simulink library "simetranss"  (R2024b)
settings: Solver=VariableStepAuto  StartTime=0.0  StopTime=10.0  RelTol=1e-3
PostLoadFcn:
  | Ts=1e-6
InitFcn:
  | Ts=1e-6
undefined symbols (not defined in the file): C, C_601, C_603, C_606, CC, Csnu, Csnubber, DiscIntNeverNeededParam, DPL, DPL1ph, FluxTable, ft2km, gcbh, h, Half, Imap2, L, L_601, L_603, L_606, Lbase, LpejoSw, Newton, R_601, R_603, R_606, Raphson, ResistanceM, Roff, Ron, RotorAngles, Rsnu, Rsnubber, Rt4, SampleTime, simetran, sps, sps_rtmsupport, StatorCurrents, T_2wind_ratio, T_Lpu, T_Lpu_pri, T_Rpu, T_Rpu_pri, T_Vpri, T_Vpri_15comp, T_Vsec, Ti, Ts_Power, Z, Zbase, Zm
libraries: fl_lib x248, ee_lib x146, nesl_utility x122, $bdroot x29, simulink x15, eeGeneralControl x2, spsStairGeneratorLib x2, artemis x1
(part 1 of 12)
Description:
  | Collection of custom SimScape real-time models.
settings Model: ModifiedByFormat=KD  Creator=Kyle Diller  LastModifiedBy=KD

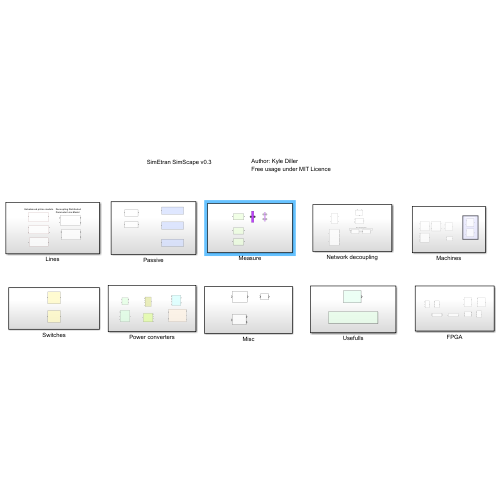
[thumbnail: Simulink's stored preview of the top-level diagram]
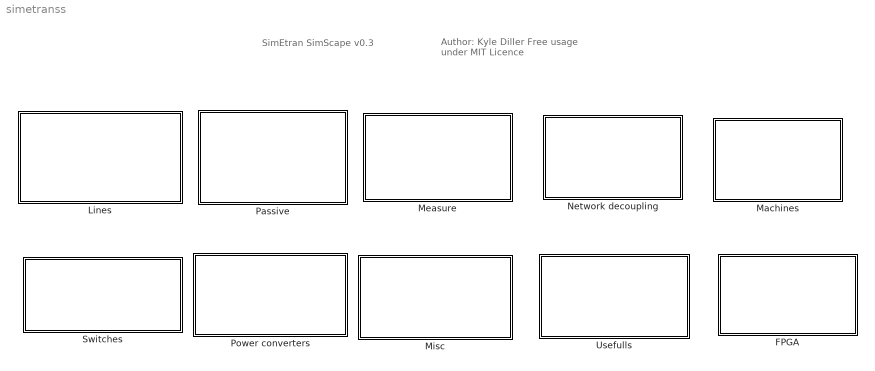
== system simetranss ==
  note: Author: Kyle Diller
      | Free usage under MIT Licence
  note: SimEtran SimScape v0.3
  FPGA : Subsystem
  Lines : Subsystem
  Machines : Subsystem
  Measure : Subsystem
  Misc : Subsystem
  Network decoupling : Subsystem
  Passive : Subsystem
  Power converters : Subsystem
  Switches : Subsystem
  Usefulls : Subsystem

== system simetranss/FPGA ==
  MATE 2-level inverter : Subsystem  mask(MATE Compensated Pejovic 2-level inverter){Lon=1e-6, Ts=Ts}
      mask prompts: Lon "Conduction state inductance (H)"; Ts "Sample time (s)"
      mask help:
      | This block implements a 2-level inverter with Pejovic switches.
      | The 2 switch are compensated at switching instant to transfer the L/C energy between the 2 switches, resulting in much better accuracy, espacially much less spurious oscillation and power losses.
      |
      | The model is design to work with no deadtime. This means that the switch gate levels must be complimentary at all time.
      | Dead-time support will come later.
  MATE 2-level inverter backup : Subsystem  mask(MATE Compensated Pejovic 2-level inverter){Lon=1e-6, Ts=Ts}
      mask prompts: Lon "Conduction state inductance (H)"; Ts "Sample time (s)"
      mask help:
      | This block implements a 2-level inverter with Pejovic switches.
      | The 2 switch are compensated at switching instant to transfer the L/C energy between the 2 switches, resulting in much better accuracy, espacially much less spurious oscillation and power losses.
      |
      | The model is design to work with no deadtime. This means that the switch gate levels must be complimentary at all time.
      | Dead-time support will come later.
  MATE 2level_Inverter SwitchingFunction(2ph) : Subsystem  mask(MATE Inverter Switching Function (2-level IGBT/Diode) (2-phase)){Ron=1e-3, Gp=250, Gi=0.1e-6, Ts=Ts, min_charge=0}
      mask prompts: Ron "Switch Ron (Ohms)"; Gp "Snubber resistance (Ohms)"; Gi "Snubber Capacitor (Ohms)"; Ts "Sample time (s)"; min_charge "Minimum rectifying current (A)"
      mask help:
      | This block implements a two-phase, 2-level inverter as a switching function.
      |
      | The block is Time-Step-Averaing capable meaning that the averaging gate ON-time is averaged at each time step.
      | With this approach, dead-times smaller than the sample time are accurately taken into account.
      |
      | The inverter can be in high impedance and rectifying states by selecting correctly the RC snubber.
      | Typically Rsnubber=L_load/Ts , then adjust Csnubber so Rsnubber*Csnubber=2*Ts.
      |
      | Minimum Rectifying current: In passive mode (no IGBT pulsing), this is the minimum rectifying current that is injected to the DC bus. This parameter is used to avoid unrealistic DC-bus charging when the inverter acts as a diode recfifier and do not impact in active control (gate pulsing) mode.
      |
      | The block has a constant admittance and is suitable for HDL coder.
  MATE 2level_Inverter SwitchingFunction(3ph) : Subsystem  mask(MATE Inverter Switching Function (2-level IGBT/Diode) (3-phase)){Ron=1e-3, Gp=250, Gi=0.1e-6, Ts=Ts, min_charge=0.1}
      mask prompts: Ron "Switch Ron (Ohms)"; Gp "Snubber resistance (Ohms)"; Gi "Snubber Capacitor (Ohms)"; Ts "Sample time (s)"; min_charge "Minimum rectifying current (A)"
      mask help:
      | This block implements a 3-phase  2-level inverter as a switching function.
      |
      | The block is Time-Step-Averaging-capable meaning that the averaging gate ON-time is averaged at each time step.
      |
      | With this approach, dead-times smaller than the sample time are accurately taken into account.
      |
      | The inverter can be in high impedance and rectifying states by selecting correctly the RC snubber.
      | Typically Rsnubber=L_load/Ts , then adjust Csnubber so Rsnubber*Csnubber=2*Ts.
      |
      | Minimum Rectifying current: In passive mode (no IGBT pulsing), this is the minimum rectifying current that is injected to the DC bus. This parameter is used to avoid unrealistic DC-bus charging when the inverter acts as a diode recfifier and do not impact in active control (gate pulsing) mode.
      |
      | The block has a constant admittance and is suitable for HDL coder.
  MATE 2level_InverterSWHIZ : Subsystem  AncestorBlock=|  mask(MATE High impedance capable Switching Function inverter (2-level IGBT/Diode)){Ron=1e-3, Gpp=10000, Gip=1e-7, Ts=Ts, min_charge=0}
      | simetranss/FPGA/MATE 2level_Inverter
      |  SwitchingFunction(2ph)
      mask prompts: Ron "Switch Ron (Ohms)"; Gpp "Snubber resistance (Ohms)"; Gip "Snubber Capacitor (Ohms)"; Ts "Sample time (s)"; min_charge "Minimum rectifying current (A)"
      mask help:
      | This block implements a two-phase, 2-level inverter as a switching function that is capable of High-impedance emulation and Averaged-time-Step-gating.
      |
      | The block is Time-Step-Averaing capable meaning that the averaging gate ON-time is averaged at each time step.
      | With this approach, dead-times smaller than the sample time are accurately taken into account.
      | Actual resolution of the inverter is only limited by the sampling of the gate values. In HIL applications, if the gate values are sampled at the FPGA clock resolution, the inverter will accurately compute the load voltage with this precision.
      |
      | The inverter can be in high impedance and rectifying states by selecting correctly the RC snubber. Note that the RC snubber is out of circuit during normal (pulsing) model of the inverter.
      | Typically Rsnubber=L_load/Ts , then adjust Csnubber so Rsnubber*Csnubber=2*Ts.
      | On FPGAs, at time step of 1 micro-seconds, R=1kOhms and C=0.1uF are often good.
      |
      | Minimum Rectifying current: In passive mode (no IGBT pulsing), this is the minimum rectifying current that is injected to the DC bus. This parameter is used to avoid unrealistic DC-bus charging when the inverter acts as a diode recfifier and do not impact in active control (gate pulsing) mode.
      |
      | The block has a constant admittance and is suitable for HDL coder.
  MATE 3levelNPC_Inverter SwitchingFunction(3ph) : Subsystem  mask(MATE Inverter Switching Function (2-level IGBT/Diode) (3-phase)){Ron=1e-3, Gp=100, Gi=0.2e-6, Ts=Ts, min_charge=0.1}
      mask prompts: Ron "Switch Ron (Ohms)"; Gp "Snubber resistance (Ohms)"; Gi "Snubber Capacitor (Ohms)"; Ts "Sample time (s)"; min_charge "Minimum rectifying current (A)"
      mask help:
      | This block implements a 3-phase  2-level inverter as a switching function.
      |
      | The block is Time-Step-Averaging-capable meaning that the averaging gate ON-time is averaged at each time step.
      |
      | With this approach, dead-times smaller than the sample time are accurately taken into account.
      |
      | The inverter can be in high impedance and rectifying states by selecting correctly the RC snubber.
      | Typically Rsnubber=L_load/Ts , then adjust Csnubber so Rsnubber*Csnubber=2*Ts.
      |
      | Minimum Rectifying current: In passive mode (no IGBT pulsing), this is the minimum rectifying current that is injected to the DC bus. This parameter is used to avoid unrealistic DC-bus charging when the inverter acts as a diode recfifier and do not impact in active control (gate pulsing) mode.
      |
      | The block has a constant admittance and is suitable for HDL coder.
  Pejovic L-C-switch component : Subsystem  mask(Pejovic Element for FPGA simulation){typ=Inductor, Lon=LpejoSw, L=L, C=C, otherSW='coming soon', Ts=Ts}
      mask prompts: typ "Element type"; Lon "Switch equivalent ON inductance (H)"; L "Inductor inductance (H)"; C "Capacitor capacitance (F)"; otherSW "Linked Compensated switch name"; Ts "Sample Time (s)"
      mask help:
      | Pejovic L-C-Switch element  in SimScape
      |
      | Implements either  an inductor, a capacitor or a switch using the Pejovic constant admittance method.
      |
      | For the Switch option, the user only has to select the equivalent ON-state inductance of the model, the corresponding Capacitance is computed internally. In the Pejovic model, Ts/Lon=Coff/Ts (Backward Euler) resulting in a constant admittance for the DAE solver.
      |
      |
      | Input signals;
      |
      | gate: the switch gate value (1 for ON , 0 for OFF) (with Switch option)
      mask init:
      | block=gcb;
      | Xcomp=0;
      | 
      | typp=get_param(block,'typ');
      | if isequal(typp,'Switch')
      |     replace_block (block ,'Followlinks' ,'on' ,'Name' ,'gate' ,'BlockType' ,'Constant' ,'Inport' ,'noprompt' ); 
      |     replace_block (block ,'Followlinks' ,'on' ,'Name' ,'init_in' ,'BlockType' ,'Inport' ,'Constant' ,'noprompt'  );
      |     replace_block (block ,'Followlinks' ,'on' ,'Name' ,'init_out' ,'BlockType' ,'Outport' ,'Terminator' ,'noprompt'  );
      |     Rsw=Lon/Ts;
      |     txt='Switch';
      | 
      | elseif isequal(typp,'Inductor')
      |     replace_block (block ,'Followlinks' ,'on' ,'Name' ,'gate' ,'BlockType' ,'Inport' ,'Constant' ,'noprompt' ); 
      |     set_param([block '/gate'],'Value','1');
      |     replace_block (block ,'Followlinks' ,'on' ,'Name' ,'init_in' ,'BlockType' ,'Inport' ,'Constant' ,'noprompt'  ); 
      |     replace_block (block ,'Followlinks' ,'on' ,'Name' ,'init_out' ,'BlockType' ,'Outport' ,'Terminator' ,'noprompt'  );
      |     Rsw=L/Ts;
      |     txt='L';
      | elseif isequal(typp,'Capacitor')
      |     replace_block (block ,'Followlinks' ,'on' ,'Name' ,'gate' ,'BlockType' ,'Inport' ,'Constant' ,'noprompt' ); 
      |     set_param([block '/gate'],'Value','0');
      |     replace_block (block ,'Followlinks' ,'on' ,'Name' ,'init_in' ,'BlockType' ,'Inport' ,'Constant' ,'noprompt'  );
      |     replace_block (block ,'Followlinks' ,'on' ,'Name' ,'init_out' ,'BlockType' ,'Outport' ,'Terminator' ,'noprompt'  );
      |     Rsw=Ts/C;
      |     txt='C';
      | elseif isequal(typp,'2-level inverter switch')
      |     replace_block (block ,'Followlinks' ,'on' ,'Name' ,'gate' ,'BlockType' ,'Constant' ,'Inport' ,'noprompt' ); 
      |     replace_block (block ,'Followlinks' ,'on' ,'Name' ,'init_in' ,'BlockType' ,'Constant' ,'Inport','noprompt'  );
      |     replace_block (block ,'Followlinks' ,'on' ,'Name' ,'init_out' ,'BlockType' ,'Terminator' ,'Outport' ,'noprompt'  );
      |     Rsw=Lon/Ts;
      |     txt='Switch half';
      |     Xcomp=1;
      | 
      | else
      | end
      | 
      | 
      | 
      | if Ts>2e-6
      |     %warndlg(['Sample Time of ' num2str(Ts) ' s. may be somehow large for the Pejovic switch to be accurate. Sample time below 2 us are recommended.'])
      | end
      mask TypeOptions typ: Switch | Inductor | Capacitor | 2-level inverter switch
      mask Display: disp(txt)
  Pejovic L/C switch : Subsystem  mask(Pejovic Switch){Lon=1e-6, Ts=Ts}
      mask prompts: Lon "Selected equivalent ON inductance (H)"; Ts "Sample Time (s)"
      mask help:
      | Pejovic switch model in SimScape
      |
      | Implements a single phase switch model using the Pejovic constant admittance method.
      | The user only has to select the equivalent ON-state inductance of the model, the corresponding Capacitance is computed internally.
      |
      | In the Pejovic model, Ts/Lon=Coff/Ts (Backward Euler) resulting in a constant admittance for the DAE solver.
      |
      | Input signals;
      |
      | gate: the switch gate value (1 for ON , 0 for OFF)
      mask init:
      | Coff=Ts*Ts/Lon;
      | Rsw=Lon/Ts;
      | 
      | if Ts>2e-6
      |     warndlg(['Sample Time of ' num2str(Ts) ' s. may be somehow large for the Pejovic switch to be accurate. Sample time below 2 us are recommended.'])
      | end
      mask Display: disp(['Pswitch'])

== system simetranss/Lines ==
  note: Unbalanced pi-line models
  note: Decoupling Distributed
      | Parameter Line Model
  Half-DPL : Subsystem  AncestorBlock=simetran/Half-DPL  mask(Simscape 3-phase Distributed Parameters Line){Phases=3, Frequency=60, Resistance=[0.01273*2 0.3864], Inductance=[0.9337e-3  4.1264e-3], Capacitance=[12.74e-9 7.751e-9], Length=75, Ts=Ts}
      mask prompts: Phases "Number of phases N"; Frequency "Frequency used for R L C specification (Hz)"; Resistance "Resistance per unit length (Ohms/km)   [N*N matrix] or [R1 R0 R0m]"; Inductance "Inductance per unit length (H/km) [N*N matrix ] or [L1 L0 L0m]"; Capacitance "Capacitance per unit length (F/km) [N*N matrix] or [C1 C0 C0m]"; Length "Line length (km)"; Ts "Sample time (s)"
      mask help:
      | Implements a 3-phases distributed parameter line (DPL) model.
      |
      | One can either specify complete [NxN] matrices or simply enter sequence parameters vectors: the  positive and zero sequence parameters for a two-phase or  three-phase transposed  line, plus the mutual zero-sequence for a  six-phase transposed  line  (2 coupled 3-phase lines).
      |
      | This DPL model allows the decoupling of computational tasks at each line ends.
      mask init:
      | % Get current block
      | currentBlock = gcb;
      | 
      | % Get electric variables
      | [Zm,R,v,Ti,to,Rt4,h,Zimp,Zmat,Yphase,ResistanceM] = ssc_dpl_cb(gcb,'funcky OpBalls', Phases, Frequency, Resistance, Inductance, Capacitance, Length);
      | 
      | delay=floor(to/Ts);
      | remd=rem(to,Ts)/Ts;
      | 
      | mess=['SimScape \n\n\n' ' DPL 3-ph'];
      mask TypeOptions Phases: 1 | 2 | 3 | 4 | 5 | 6 | 8 | 9 | 10 | 12
      mask Display:
      | plot(0,0,100,100,[20,20,80,80,80,80,20,20,10],[50,40,40,50,50,61,61,50,50])
      | disp('half-DPL 3ph)')
      | %disp(mess)
  Half-DPL1ph : Subsystem  AncestorBlock=simetran/Half-DPL1ph  mask(Simscape 1-phase Distributed Parameters Line){Phases=1, Frequency=60, Resistance=0.015, Inductance=0.792e-3, Capacitance=14.4e-9, Length=300, Ts=Ts, cd=on}
      mask prompts: Phases "Number of phases N"; Frequency "Frequency used for R L C specification (Hz)"; Resistance "Resistance per unit length (Ohms/km)   [N*N matrix] or [R1 R0 R0m]"; Inductance "Inductance per unit length (H/km) [N*N matrix ] or [L1 L0 L0m]"; Capacitance "Capacitance per unit length (F/km) [N*N matrix] or [C1 C0 C0m]"; Length "Line length (km)"; Ts "Sample time (s)"; cd "Compensate for explicit Unit Delay of propagation"
      mask help:
      | Implements a single-phase distributed parameter line (DPL) model.
      |
      | This DPL model allows the decoupling of computational tasks at each line ends.
      |
      | In SimScape with concurrent (parallel) task simulation, one may be forced to add an explicit and external one-step delay at the propagation input of the line. In this case, the option 'Compensate for explicit Unit Delay of propagation' will exactly compensate this external delay.
      mask init:
      | % Get current block
      | currentBlock = gcb;
      | 
      | % Get electric variables
      | [Zm,R,v,Ti,to,Rt4,h,Zimp,Zmat,Yphase,ResistanceM] = ssc_dpl_cb(gcb,'variable_mask_maskinitialization', Phases, Frequency, Resistance, Inductance, Capacitance, Length);
      | % nphase=Phases;
      | % [Zm,R,v,Ti]=powericon('Distributed Parameter Line Model',nphase,Frequency,Resistance,Inductance,Capacitance);
      | %         %[Zmxx,Rmxx,Smodexx,Tixx] = blmodlin(nphase,Frequency,Resistance,Inductance,Capacitance);
      | %         %warning(w);
      | % 
      | % 
      | %         to = Length ./ v;
      | %         Rt4 = R * Length / 4;
      | %         h = (Zm - Rt4) ./ (Zm + Rt4);
      | %         Zimp = Zm + Rt4;
      | % 
      | %         % Calculate Zmat
      | %         Zmat = zeros(nphase);
      | %         for t = 1 : nphase
      | %             Zmat(t,t) = Zimp(t);
      | %         end
      | % 
      | %         % Calculate Y phase
      | %         Yphase=Ti*inv(Zmat)*(Ti');
      | % 
      | %         % Calculate R_x_0
      | %         ResistanceM = zeros(nphase);
      | %         for t = 1 : nphase
      | %             ResistanceM(t,t) = 1/(sum(Yphase(t,1:nphase)));
      | %         end
      | % 
      | %         % Calculate R_m_n
      | %         for t = 1 : nphase
      | %             for u = t+1: nphase
      | %                 ResistanceM(t,u) = -1/(Yphase(u,t));
      | %             end
      | %         end
      | V1_init=[0 zeros(1,Phases); 0.1 zeros(1,Phases)];
      | delay=floor(to/Ts);
      | if cd==1
      |     delay=delay-1;
      | end
      | if delay<1
      |     error('Line delay is less than 1 time step');
      | end
      | remd=rem(to,Ts)/Ts;
      mask TypeOptions Phases: 1 | 2 | 3 | 4 | 5 | 6 | 8 | 9 | 10 | 12
      mask Display:
      | plot(0,0,100,100,[20,20,80,80,80,80,20,20,10],[50,40,40,50,50,61,61,50,50])
      | disp('half-DPL 1ph)')
      | %disp(mess)
  mate_1ph_piline : Subsystem  mask(Unbalanced 1-phase pi-line (IEEE 123 node)){FF=60, conf=config 9, lenfeet=1500, dmi=off, RR1=0.8, LL1=0.002, CC1=7e-9, lenkm=300*ft2km}
      mask prompts: FF "Nominal frequency (Hz)"; conf "IEEE 123 node line configuration"; lenfeet "Length (ft)"; dmi "Direct RLC matrix input"; RR1 "Resistance (Ohms/km)"; LL1 "Inductance (H/km)"; CC1 "Capacitance (F/km)"; lenkm "Line length (km)"
      mask help: This model uses the comfiguration of the IEEE 123 node standard.
      mask init:
      | freq=str2num(get_param(gcb,'FF'));
      | choix=get_param(gcb,'conf');
      |  ch=choix(8:end);
      |  confnum=str2num(ch);
      | 
      |  if isequal(get_param(gcb,'dmi'),'off')
      | 
      |  lenstr=get_param(gcb, 'lenfeet');
      | % IEEE 123 bus
      | 
      | % miles/km
      | mi2km = 1.609344;
      | % feet to km
      | ft2km = 0.0003048;
      | % microsiemens to Farads
      | ms2F = 1/2/pi/freq*1e-6;
      | % ohms to Henry
      | x2H=1/2/pi/freq;
      | 
      | % lenght in km
      | len=lenfeet*ft2km;
      | 
      | %% Configuration 9 - series reactance - ohm/mile [A]
      | 
      | lineData(9).R = 1.3292;
      |     
      | lineData(9).X = 1.3475;
      | 
      | % charging susceptance - microsiemens/mile
      | 
      | lineData(9).B = 4.5193;
      | 
      | 
      | 
      | %% Configuration 10 - series reactance - ohm/mile [B]
      | 
      | lineData(10).R = 1.3292;
      |     
      | lineData(10).X = 1.3475;
      | 
      | % charging susceptance - microsiemens/mile
      | 
      | lineData(10).B = 4.5193;
      | 
      | 
      | 
      | %% Configuration 11 - series reactance - ohm/mile [C]
      | 
      | lineData(11).R = 1.3292;
      |     
      | lineData(11).X = 1.3475;
      | 
      | % charging susceptance - microsiemens/mile
      | 
      | lineData(11).B = 4.5193;
      | 
      | 
      |     %convert for SPS
      | 
      | RR = (lineData(confnum).R)/mi2km;
      | 
      | LL = (lineData(confnum).X)/mi2km*x2H;
      | 
      | CC = (lineData(confnum).B)/mi2km*ms2F;  % len variable moved to underlying RLC componants
      | 
      | C11=CC/2;
      | 
      | mess=['MATE IEEE-123node \n\n\n' choix '  ' lenstr ' ft (1ph)'];
      | 
      |  else
      | 
      |     RR=RR1;
      |     LL=LL1;
      |     CC=CC1;
      |     
      |     C11=CC/2;
      |     len=lenkm;
      |     mess=['MATE \n\n\n' num2str(lenkm) ' km'];
      |  end
      mask TypeOptions conf: config 9 | config 10 | config 11
      mask Callback dmi:
      | block = gcb;
      | type=get_param(block,'dmi');
      | 
      | visib=get_param(block,'MaskVisibilities');
      | visib{4}='on';
      | if isequal(type,'on')
      |     visib{1}='off';;visib{2}='off';visib{3}='off';visib{5}='on';visib{6}='on';visib{7}='on';visib{8}='on';
      | else
      |     visib{1}='on';;visib{2}='on';visib{3}='on';visib{5}='off';visib{6}='off';visib{7}='off';visib{8}='off';
      | end
      | set_param(block,'MaskVisibilities',visib);
      mask Display:
      | plot(0,0,100,100,[20,20,80,80,90,80,80,20,20,10],[50,40,40,50,50,50,61,61,50,50],[56,39],[55,55],[44,44],[44,55],[53,50,50],[44,48,55])
      | disp(mess)
  mate_2ph_piline : Subsystem  mask(Unbalanced 3-phase pi-line (IEEE 123 node)){FF=60, conf=config 7, lenfeet=300, dmi=off, RR22=R_603(2:3,2:3), LL22=L_603(2:3,2:3), CC22=C_603(2:3,2:3), lenkm=500*ft2km}
      mask prompts: FF "Nominal frequency (Hz)"; conf "IEEE 123 node line configuration"; lenfeet "Length (ft)"; dmi "Direct RLC matrix input"; RR22 "Resistance (Ohms/km)"; LL22 "Inductance (H/km)"; CC22 "Capacitance (F/km)"; lenkm "Line length (km)"
      mask help: This model uses the comfiguration of the IEEE 123 node standard.
      mask init:
      | freq=str2num(get_param(gcb,'FF'));
      | choix=get_param(gcb,'conf');
      | ch=choix(8:end);
      | confnum=str2num(ch);
      | 
      | if isequal(get_param(gcb,'dmi'),'off')
      | 
      | lenstr=get_param(gcb, 'lenfeet');
      | 
      | % IEEE 123 bus
      | 
      | % miles/km
      | mi2km = 1.609344;
      | % feet to km
      | ft2km = 0.0003048;
      | % microsiemens to Farads
      | ms2F = 1/2/pi/freq*1e-6;
      | % ohms to Henry
      | x2H=1/2/pi/freq;
      | 
      | % lenght in km
      | len=lenfeet*ft2km;
      | 
      | %% Configuration 7 - series reactance - ohm/mile [A,C]
      | 
      | lineData(7).R = [ 0.4576 0.1535
      |         0.1535 0.4615];
      |     
      | lineData(7).X = [ 1.0780 0.3849
      |         0.3849 1.0651];
      | 
      | % charging susceptance - microsiemens/mile
      | 
      | lineData(7).B = [ 5.1154  -1.0549
      |         -1.0549 5.1704];
      | 
      | 
      | 
      | %% Configuration 8 - series reactance - ohm/mile [A,B]
      | 
      | lineData(8).R = [ 0.4576 0.1535
      |         0.1535 0.4615];
      |     
      | lineData(8).X = [ 1.0780 0.3849
      |         0.3849 1.0651];
      | 
      | % charging susceptance - microsiemens/mile
      | 
      | lineData(8).B = [ 5.1154  -1.0549
      |         -1.0549  5.1704];
      | 
      |     %convert for SPS
      | 
      | RR = (lineData(confnum).R)/mi2km;
      | 
      | LL = (lineData(confnum).X)/mi2km*x2H;
      | 
      | CC = (lineData(confnum).B)/mi2km*ms2F;  % len variable moved to the componant parameter
      | 
      | 
      | C11=sum(CC(1,:));
      | C22=sum(CC(2,:));
      | 
      | C12=-CC(1,2);
      | 
      | mess=['MATE IEEE-123node \n\n\n' choix '  ' lenstr ' ft (2ph)'];
      | 
      | else
      |     RR=RR22;
      |     LL=LL22;
      |     CC=CC22;
      |     
      |     C11=sum(CC(1,:));
      |     C22=sum(CC(2,:));
      |     C12=-CC(1,2);
      |     len=lenkm;
      |     mess=['MATE \n\n\n' num2str(lenkm) ' km'];
      | 
      | end
      mask TypeOptions conf: config 7 | config 8
      mask Callback dmi:
      | block = gcb;
      | type=get_param(block,'dmi');
      | 
      | visib=get_param(block,'MaskVisibilities');
      | visib{4}='on';
      | if isequal(type,'on')
      |     visib{1}='off';;visib{2}='off';visib{3}='off';visib{5}='on';visib{6}='on';visib{7}='on';visib{8}='on';
      | else
      |     visib{1}='on';;visib{2}='on';visib{3}='on';visib{5}='off';visib{6}='off';visib{7}='off';visib{8}='off';
      | end
      | set_param(block,'MaskVisibilities',visib);
      mask Display:
      | plot(0,0,100,100,[20,20,80,80,90,80,80,20,20,10],[50,40,40,50,50,50,61,61,50,50],[56,39],[55,55],[44,44],[44,55],[53,50,50],[44,48,55])
      | disp(mess)
  mate_3ph_piline : Subsystem  mask(MATE Unbalanced 3-phase pi-line (IEEE 123 node)){FF=60, conf=config 6, lenfeet=2500, dmi=off, RR33=R_606, LL33=L_606, CC33=C_606, lenkm=500*ft2km}
      mask prompts: FF "Nominal frequency (Hz)"; conf "IEEE 123 node line configuration"; lenfeet "Length (ft)"; dmi "Direct RLC matrix input"; RR33 "Resistance (Ohms/km)"; LL33 "Inductance (H/km)"; CC33 "Capacitance (F/km)"; lenkm "Line length (km)"
      mask help:
      | This model uses the line configurations of the IEEE 123 node standard.
      | Alternatively, the user can enter the RLC matrices of the line.
      |
      | Note: the Simscape 3-phase mutual inductance does not permit matrix mutual resistance and therefore introduce an error in 3-phase unbalanced pi-line models.
      mask init:
      | freq=str2num(get_param(gcb,'FF'));
      | choix=get_param(gcb,'conf');
      | ch=choix(8:end);
      | confnum=str2num(ch);
      | 
      | if isequal(get_param(gcb,'dmi'),'off')
      | 
      | lenstr=get_param(gcb,'lenfeet');
      | 
      | % IEEE 123 bus 
      | 
      | % miles/km
      | mi2km = 1.609344;
      | % feet to km
      | ft2km = 0.0003048;
      | % microsiemens to Farads
      | ms2F = 1/2/pi/freq*1e-6;
      | % ohms to Henry
      | x2H=1/2/pi/freq;
      | 
      | % lenght in km
      | len=lenfeet*ft2km;
      | 
      | %% Configuration 1 - series reactance - ohm/mile
      | 
      | lineData(1).R = [ 0.4576 0.1560 0.1535
      |         0.1560 0.4666 0.1580
      |         0.1535 0.1580 0.4615];
      |     
      | lineData(1).X = [ 1.0780 0.5017 0.3849
      |         0.5017 1.0482 0.4236
      |         0.3849 0.4236 1.0651];
      | 
      | % charging susceptance - microsiemens/mile
      | 
      | lineData(1).B = [ 5.6765 -1.8319 -0.6982
      |         -1.8319 5.9809 -1.1645
      |         -0.6982 -1.1645 5.3971];
      | 
      | 
      | 
      | %% Configuration 2 - series reactance - ohm/mile
      | 
      | lineData(2).R = [ 0.4666 0.1580 0.1560
      |         0.1580 0.4615 0.1535
      |         0.1560 0.1535 0.4576];
      |     
      | lineData(2).X = [ 1.0482 0.4236 0.5017
      |         0.4236 1.0651 0.3849
      |         0.5017 0.3849 1.0780];
      | 
      | % charging susceptance - microsiemens/mile
      | 
      | lineData(2).B = [ 5.9809 -1.1645 -1.8319
      |         -1.1645 5.3971 -0.6982
      |         -1.8319 -0.6982 5.6765];
      | 
      | 
      | %% Configuration 3 - series reactance - ohm/mile
      | 
      | lineData(3).R = [ 0.4615 0.1535 0.1580
      |         0.1535 0.4576 0.1560
      |         0.1580 0.1560 0.4666];
      |     
      | lineData(3).X = [ 1.0651 0.3849 0.4236
      |         0.3849 1.0780 0.5017
      |         0.4236 0.5017 1.0482];
      | 
      | % charging susceptance - microsiemens/mile
      | 
      | lineData(3).B = [ 5.3971 -0.6982 -1.1645
      |         -0.6982 5.6765 -1.8319
      |         -1.1645 -1.8319 5.9809];
      | 
      | 
      | %% Configuration 4 - series reactance - ohm/mile
      | 
      | lineData(4).R = [ 0.4615 0.1580 0.1535
      |         0.1580 0.4666 0.1560
      |         0.1535 0.1560 0.4576];
      |     
      | lineData(4).X = [ 1.0651 0.4236 0.3849
      |         0.4236 1.0482 0.5017
      |         0.3849 0.5017 1.0780];
      | 
      | % charging susceptance - microsiemens/mile
      | 
      | lineData(4).B = [ 5.3971 -1.1645 -0.6982
      |         -1.1645 5.9809 -1.8319
      |         -0.6982 -1.8319 5.6765];
      | 
      | 
      | %% Configuration 5 - series reactance - ohm/mile
      | 
      | lineData(5).R = [ 0.4666 0.1560 0.1580
      |         0.1560 0.4576 0.1535
      |         0.1580 0.1535 0.4615];
      |     
      | lineData(5).X = [ 1.0482 0.5017 0.4236
      |         0.5017 1.0780 0.3849
      |         0.4236 0.3849 1.0651];
      | 
      | % charging susceptance - microsiemens/mile
      | 
      | lineData(5).B = [ 5.9809 -1.8319 -1.1645
      |         -1.8319 5.6765 -0.6982
      |         -1.1645 -0.6982 5.3971];
      | 
      | 
      | %% Configuration 6 - series reactance - ohm/mile
      | 
      | lineData(6).R = [ 0.4576 0.1535 0.1560
      |         0.1535 0.4615 0.1580
      |         0.1560 0.1580 0.4666];
      |     
      | lineData(6).X = [ 1.0780 0.3849 0.5017
      |         0.3849 1.0651 0.4236
      |         0.5017 0.4236 1.0482];
      | 
      | % charging susceptance - microsiemens/mile
      | 
      | lineData(6).B = [ 5.6765 -0.6982 -1.8319
      |         -0.6982 5.3971 -1.1645
      |         -1.8319 -1.1645 5.9809];
      |     
      | %% Configuration 12 - series reactance - ohm/mile
      | 
      | lineData(12).R = [1.5209 0.5198 0.4924
      |         0.5198 1.5329 0.5198
      |         0.4924 0.5198 1.5209];
      |     
      | lineData(12).X = [0.7521 0.2775 0.2157
      |         0.2775 0.7162 0.2775
      |         0.2157 0.2775 0.7521];
      | 
      | % charging susceptance - microsiemens/mile
      | 
      | lineData(12).B = [67.2242 -1e-6   -1e-6
      |         -1e-6    67.2242 -1e-6
      |         -1e-6    -1e-6   67.2242];
      | 
      | %convert for SPS
      | 
      | RR = (lineData(confnum).R)/mi2km; % note len variable moved into the componant parameters
      | 
      | LL = (lineData(confnum).X)/mi2km*x2H; % note len variable moved into the componant parameters
      | 
      | CC = (lineData(confnum).B)/mi2km*ms2F;  % note len variable moved into the componant parameters
      | 
      | C11=sum(CC(1,:));
      | C22=sum(CC(2,:));
      | C33=sum(CC(3,:));
      | C12=-CC(1,2);
      | C13=-CC(1,3);
      | C23=-CC(2,3);
      | mess=['MATE IEEE-123node \n\n\n' choix '  ' lenstr ' ft (3ph)' ];
      | 
      | 
      | else
      |     RR=RR33;
      |     LL=LL33;
      |     CC=CC33;
      |     len=lenkm;
      |     C11=sum(CC(1,:));
      |     C22=sum(CC(2,:));
      |     C33=sum(CC(3,:));
      |     C12=-CC(1,2);
      |     C13=-CC(1,3);
      |     C23=-CC(2,3);
      |     mess=['MATE \n\n\n' num2str(lenkm) ' km'];
      | end
      | 
      | %warning('the Simscape 3-phase mutual inductance does not permit matrix mutual resistance and therefore introduce an error in 3-phase pi-line models')
      mask TypeOptions conf: config 1 | config 2 | config 3 | config 4 | config 5 | config 6 | config 12
      mask Callback dmi:
      | block = gcb;
      | type=get_param(block,'dmi');
      | 
      | visib=get_param(block,'MaskVisibilities');
      | visib{4}='on';
      | if isequal(type,'on')
      |     visib{1}='off';;visib{2}='off';visib{3}='off';visib{5}='on';visib{6}='on';visib{7}='on';visib{8}='on';
      | else
      |     visib{1}='on';;visib{2}='on';visib{3}='on';visib{5}='off';visib{6}='off';visib{7}='off';visib{8}='off';
      | end
      | set_param(block,'MaskVisibilities',visib);
      mask Display:
      | plot(0,0,100,100,[20,20,80,80,90,80,80,20,20,10],[50,40,40,50,50,50,61,61,50,50],[56,39],[55,55],[44,44],[44,55],[53,50,50],[44,48,55])
      | disp(mess)
